simulink model "PIDModeloPlantaBuenazo"  (R2016a)
settings: Solver=ode45  StartTime=0.0  StopTime=10  MaxStep=0.01  RelTol=1e-3
libraries: simulink x1
settings Model: Creator=i95sa  LastModifiedBy=i95sa
settings DataIOCC: SaveFormat=StructureWithTime
settings DebuggingCC: FcnCallInpInsideContextMsg=EnableAllAsWarning
settings HardwareCC: ProdWordSize=32  ProdHWDeviceType=Specified
settings ConfigComp: CovSFcnEnable=off

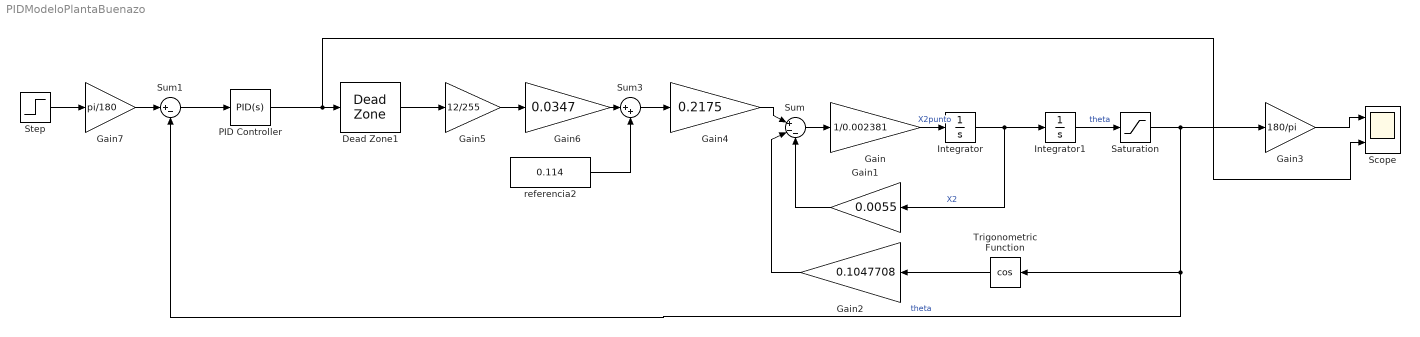
== system PIDModeloPlantaBuenazo ==
  Dead Zone1 : DeadZone  LowerValue=0  UpperValue=0  SaturateOnIntegerOverflow=on
  Gain : Gain  Gain=1/0.002381
  Gain1 : Gain  Gain=0.0055
  Gain2 : Gain  Gain=0.1047708
  Gain3 : Gain  Gain=180/pi
  Gain4 : Gain  Gain=0.2175
  Gain5 : Gain  Gain=12/255
  Gain6 : Gain  Gain=0.0347
  Gain7 : Gain  Gain=pi/180
  Integrator : Integrator
  Integrator1 : Integrator  InitialCondition=-0.65
  PID Controller : simulink/Continuous/PID Controller  Controller=PID  TimeDomain=Continuous-time  SampleTime=-1  IntegratorMethod=Forward Euler  FilterMethod=Forward Euler  Form=Parallel  UseFilter=on  ControllerParametersSource=internal  P=10  I=1  D=0.01  N=100  InitialConditionSource=internal  InitialConditionForIntegrator=0  InitialConditionForFilter=0  ExternalReset=none  LimitOutput=on  UpperSaturationLimit=255  LowerSaturationLimit=-20  LinearizeAsGain=off  AntiWindupMode=clamping  Kb=1  TrackingMode=off  Kt=1  PParamMin=[]  PParamMax=[]  IParamMin=[]  IParamMax=[]  DParamMin=[]  DParamMax=[]  NParamMin=[]  NParamMax=[]  KbParamMin=[]  KbParamMax=[]  KtParamMin=[]  KtParamMax=[]  POutMin=[]  POutMax=[]  IOutMin=[]  IOutMax=[]  DOutMin=[]  DOutMax=[]  NOutMin=[]  NOutMax=[]  KbOutMin=[]  KbOutMax=[]  KtOutMin=[]  KtOutMax=[]  IntegratorOutMin=[]  IntegratorOutMax=[]  FilterOutMin=[]  FilterOutMax=[]  SumOutMin=[]  SumOutMax=[]  SumI1OutMin=[]  SumI1OutMax=[]  SumI2OutMin=[]  SumI2OutMax=[]  SumI3OutMin=[]  SumI3OutMax=[]  SumDOutMin=[]  SumDOutMax=[]  SaturationOutMin=[]  SaturationOutMax=[]  IntegratorContinuousStateAttributes=''  IntegratorStateMustResolveToSignalObject=off  IntegratorRTWStateStorageClass=Auto  FilterContinuousStateAttributes=''  FilterStateMustResolveToSignalObject=off  FilterRTWStateStorageClass=Auto  DifferentiatorICPrevScaledInput=0  DifferentiatorOutMin=[]  DifferentiatorOutMax=[]
  Saturation : Saturate  UpperLimit=0.65  LowerLimit=-0.65
  Scope : Scope  NumInputPorts=2
  Step : Step  Time=0  After=0  SampleTime=0
  Sum : Sum  Inputs=|+--
  Sum1 : Sum  Inputs=|+-
  Sum3 : Sum  Inputs=|++
  Trigonometric Function : Trigonometry  Operator=cos
  referencia2 : Constant  Value=0.114
  wires:
  Sum/1 -> Gain/1
  Gain/1 -> Integrator/1  "X2punto"
  Integrator/1 -> Integrator1/1, Gain1/1  "X2"
  Trigonometric Function/1 -> Gain2/1
  Gain1/1 -> Sum/3
  Integrator1/1 -> Saturation/1  "theta"
  Gain2/1 -> Sum/2
  Gain4/1 -> Sum/1
  referencia2/1 -> Sum3/2
  Sum3/1 -> Gain4/1
  Gain5/1 -> Gain6/1
  Gain6/1 -> Sum3/1
  Dead Zone1/1 -> Gain5/1
  Sum1/1 -> PID Controller/1
  Step/1 -> Gain7/1
  PID Controller/1 -> Scope/2, Dead Zone1/1
  Gain3/1 -> Scope/1
  Gain7/1 -> Sum1/1
  Saturation/1 -> Sum1/2, Trigonometric Function/1, Gain3/1  "theta"
